simulink subsystem "RotateTransform"  (R2020b)
settings: Solver=VariableStepAuto  StartTime=0.0  StopTime=10.0  RelTol=1e-3
settings Model: Creator=tomonori  LastModifiedBy=tomonori

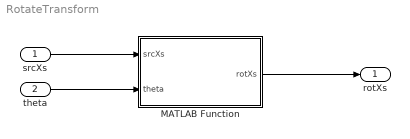
== system RotateTransform ==
  srcXs : Inport
  theta : Inport  Port=2
  MATLAB Function : MATLAB Function  TreatAsAtomicUnit=on
  rotXs : Outport
  wires:
  theta/1 -> MATLAB Function/2(theta)
  srcXs/1 -> MATLAB Function/1(srcXs)
  MATLAB Function/1(rotXs) -> rotXs/1

== matlab function RotateTransform/MATLAB Function ==
  data: srcXs input; rotXs output; theta input
function rotXs = Rotation(srcXs, theta)

%{
     cos -sin | x  =  nx
     sin  cos | y     ny
     2 * 2 , 2 * 1 : 2 * 1
     
     cos -sin | x1 x2 ... xN  =  nx1 nx2 ... nxN
     sin  cos | y1 y2 ... yN     ny1 ny2 ... nyN
     2 * 2 , 2 * N : 2 * N
     
     (x1 x2 ... xN)^T | (cos -sin)^T  =  (nx1 nx2 ... nxN)^T
     (y1 y2 ... yN)   | (sin  cos)       (ny1 ny2 ... nyN)
     N * 2 , 2 * 2 : N * 2
%}

R = [cos(theta), -sin(theta);
     sin(theta), cos(theta)];

rotXs = srcXs * R';
